simulink model "num2"  (R2019a)
settings: Solver=VariableStepAuto  StartTime=0.0  StopTime=10.0  RelTol=1e-3
undefined symbols (not defined in the file): A, B, C
settings Model: Creator=julia  LastModifiedBy=julia

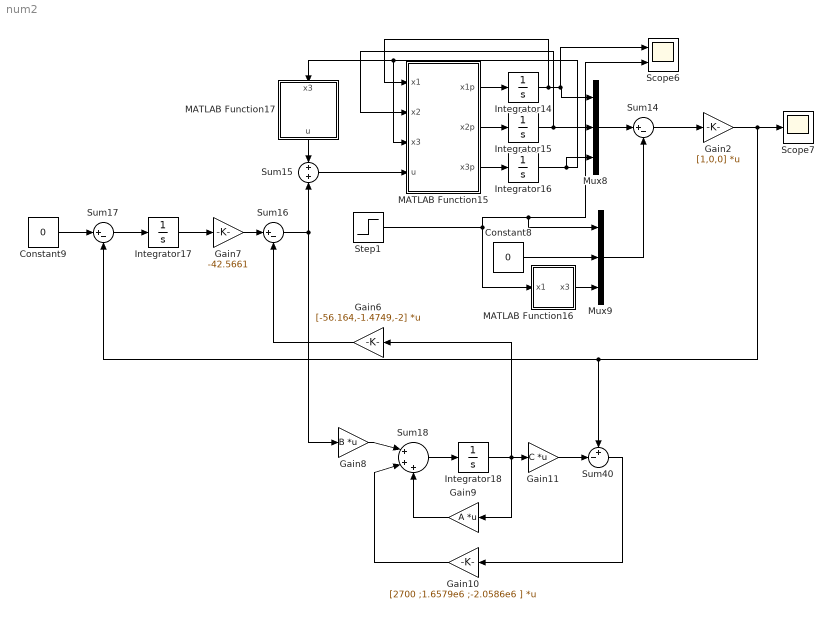
== system num2 ==
  Constant8 : Constant  Value=0
  Constant9 : Constant  Value=0
  Gain10 : Gain  Gain=[2700 ;1.6579e6 ;-2.0586e6 ]  Multiplication=Matrix(K*u)
  Gain11 : Gain  Gain=C  Multiplication=Matrix(K*u)
  Gain2 : Gain  Gain=[1,0,0]  Multiplication=Matrix(K*u)
  Gain6 : Gain  Gain=[-56.164,-1.4749,-2]  Multiplication=Matrix(K*u)
  Gain7 : Gain  Gain=-42.5661
  Gain8 : Gain  Gain=B  Multiplication=Matrix(K*u)
  Gain9 : Gain  Gain=A  Multiplication=Matrix(K*u)
  Integrator14 : Integrator  InitialCondition=5e-3
  Integrator{15..18} (4 alike) : Integrator
  MATLAB Function15 : MATLAB Function  TreatAsAtomicUnit=on
  MATLAB Function16 : MATLAB Function  TreatAsAtomicUnit=on
  MATLAB Function17 : MATLAB Function  TreatAsAtomicUnit=on
  Mux8 : Mux  Inputs=3
  Mux9 : Mux  Inputs=3
  Scope6 : Scope  NumInputPorts=2
  Scope7 : Scope
  Step1 : Step  Time=0  Before=5e-3  After=10e-3  SampleTime=0
  Sum14 : Sum  Inputs=|+-
  Sum15 : Sum  Inputs=+|+
  Sum16 : Sum  Inputs=|+-
  Sum17 : Sum  Inputs=|+-
  Sum18 : Sum  Inputs=|+++
  Sum40 : Sum  Inputs=+-|
  wires:
  Sum40/1 -> Gain10/1
  Gain11/1 -> Sum40/2
  Integrator18/1 -> Gain11/1, Gain9/1, Gain6/1
  Sum18/1 -> Integrator18/1
  Gain10/1 -> Sum18/2
  Gain9/1 -> Sum18/3
  Gain8/1 -> Sum18/1
  MATLAB Function15/1(x1p) -> Integrator14/1
  MATLAB Function15/2(x2p) -> Integrator15/1
  MATLAB Function15/3(x3p) -> Integrator16/1
  Integrator14/1 -> MATLAB Function15/1(x1), Scope6/1, Mux8/1
  Integrator15/1 -> MATLAB Function15/2(x2), Mux8/2
  Integrator16/1 -> MATLAB Function17/1(x3), MATLAB Function15/3(x3), Mux8/3
  Mux8/1 -> Sum14/1
  Constant8/1 -> Mux9/2
  Step1/1 -> MATLAB Function16/1(x1), Scope6/2, Mux9/1
  MATLAB Function16/1(x3) -> Mux9/3
  Mux9/1 -> Sum14/2
  Sum15/1 -> MATLAB Function15/4(u)
  MATLAB Function17/1(u) -> Sum15/1
  Gain7/1 -> Sum16/1
  Sum17/1 -> Integrator17/1
  Sum16/1 -> Gain8/1, Sum15/2
  Sum14/1 -> Gain2/1
  Gain2/1 -> Scope7/1, Sum40/1, Sum17/2
  Constant9/1 -> Sum17/1
  Integrator17/1 -> Gain7/1
  Gain6/1 -> Sum16/2

== matlab function num2/MATLAB Function15 ==
  data: x1 input size=1; x1p output size=1; x2 input size=1; x3 input size=1; x2p output size=1; x3p output size=1; u input size=1
function [x1p,x2p,x3p] = planta(x1,x2,x3,u)
c=0.1;
m=0.01;
L=100e-3;
r=10;
g=9.81;

x1p=x2;
x2p=g-(c/m)*((x3^2)/x1);
x3p=-(r/L)*x3+(1/L)*u;

== matlab function num2/MATLAB Function16 ==
  data: x1 input size=1; x3 output size=1
function x3  = fcn(x1)
c=1
m=0.1
L=0.01
r=1
g=9.81

x3=sqrt((m*g*x1)/c);

== matlab function num2/MATLAB Function17 ==
  data: x3 input size=1; u output size=1
function u  = u(x3)
c=1
m=0.1
L=0.01
r=1
g=9.81

u=r*x3;
